simulink model "LaengsDynamicModell"  (R2018b)
settings: Solver=VariableStepAuto  StartTime=0.0  StopTime=10.0  RelTol=1e-3
model workspace (MAT data in the model file):
  g = 9.81
  hs = 0.5
  l = 2.8
  lv = 1.344
  rBreakPoints = [0 0.25 1]
  rBreakpoints = [0 0.25 1]
  rTableData = [0 1 1]
  v0 = 19.4444444444
  zBreakpoints = [0 1.5 1.95 2.15 10]
  zTableData = [0 0 0.1 1 1]
  zh_z = 1
  zv_z = 1
libraries: simulink x3
settings Model: Creator=User  LastModifiedBy=gregoryseibert

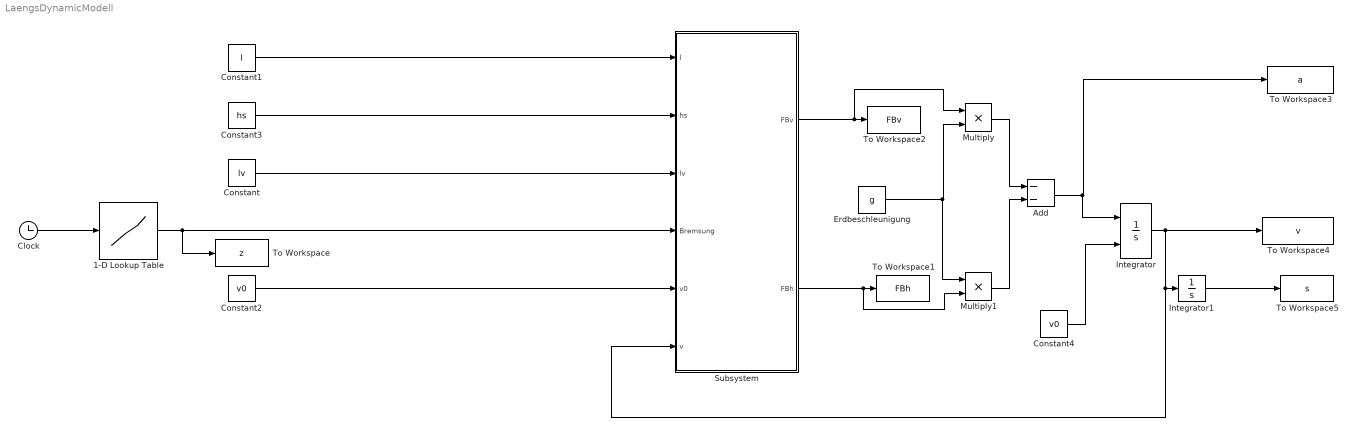
== system LaengsDynamicModell ==
  1-D Lookup Table : Lookup_n-D  NumberOfTableDimensions=1  BreakpointsForDimension1=zBreakpoints  Table=zTableData  InternalRulePriority=Speed  RndMeth=Simplest  InputSameDT=on
  Add : Sum  Inputs=--
  Clock : Clock
  Constant : Constant  Value=lv
  Constant1 : Constant  Value=l
  Constant2 : Constant  Value=v0
  Constant3 : Constant  Value=hs
  Constant4 : Constant  Value=v0
  "Erdbeschleunigung " : Constant  Value=g
  Integrator : Integrator  InitialConditionSource=external  LimitOutput=on  LowerSaturationLimit=0
  Integrator1 : Integrator
  Multiply : Product
  Multiply1 : Product
  Subsystem : Subsystem
  To Workspace : ToWorkspace  VariableName=z  SaveFormat=Timeseries  SampleTime=-1
  To Workspace1 : ToWorkspace  VariableName=FBh  SaveFormat=Timeseries  SampleTime=-1
  To Workspace2 : ToWorkspace  VariableName=FBv  SaveFormat=Timeseries  SampleTime=-1
  To Workspace3 : ToWorkspace  VariableName=a  SaveFormat=Timeseries  SampleTime=-1
  To Workspace4 : ToWorkspace  VariableName=v  SaveFormat=Timeseries  SampleTime=-1
  To Workspace5 : ToWorkspace  VariableName=s  SaveFormat=Timeseries  SampleTime=-1
  wires:
  Clock/1 -> 1-D Lookup Table/1
  1-D Lookup Table/1 -> Subsystem/4("Bremsung "), To Workspace/1
  Constant1/1 -> Subsystem/1("l ")
  Constant3/1 -> Subsystem/2(hs)
  Constant/1 -> Subsystem/3(lv)
  Constant2/1 -> Subsystem/5("v0 ")
  Subsystem/1(FBv) -> Multiply/1, To Workspace2/1
  Subsystem/2(FBh) -> Multiply1/2, To Workspace1/1
  "Erdbeschleunigung "/1 -> Multiply1/1, Multiply/2
  Multiply/1 -> Add/1
  Multiply1/1 -> Add/2
  Add/1 -> Integrator/1, To Workspace3/1
  Constant4/1 -> Integrator/2
  Integrator/1 -> Subsystem/6("v "), Integrator1/1, To Workspace4/1
  Integrator1/1 -> To Workspace5/1

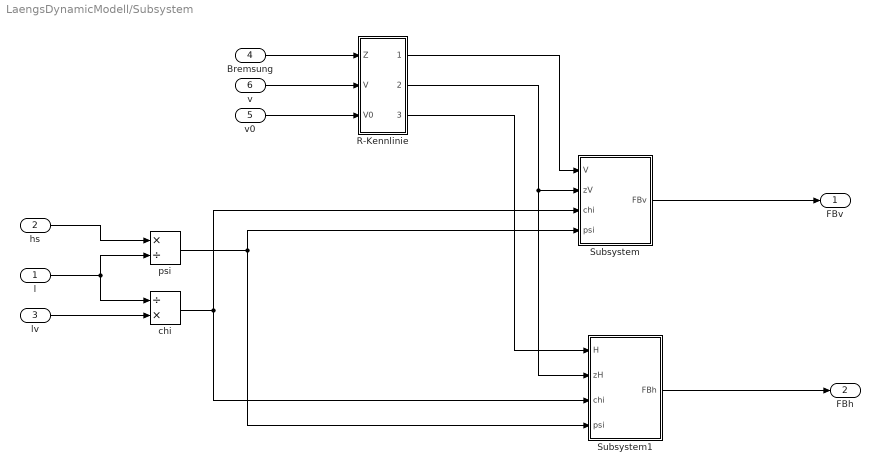
== system LaengsDynamicModell/Subsystem ==
  "l " : Inport
  hs : Inport  Port=2
  lv : Inport  Port=3
  "Bremsung " : Inport  Port=4
  "v0 " : Inport  Port=5
  "v " : Inport  Port=6
  R-Kennlinie : Subsystem
  Subsystem : Subsystem
  Subsystem1 : Subsystem
  chi : Product  Inputs=/*
  psi : Product  Inputs=*/
  FBv : Outport
  FBh : Outport  Port=2
  wires:
  "l "/1 -> chi/1, psi/2
  hs/1 -> psi/1
  lv/1 -> chi/2
  "Bremsung "/1 -> R-Kennlinie/1(Z)
  "v "/1 -> R-Kennlinie/2(V)
  "v0 "/1 -> R-Kennlinie/3("V0 ")
  psi/1 -> Subsystem/4(psi), Subsystem1/4(psi)
  chi/1 -> Subsystem/3(chi), Subsystem1/3(chi)
  R-Kennlinie/2("zOut ") -> Subsystem1/2(zH), Subsystem/2(zV)
  R-Kennlinie/3(hOut) -> Subsystem1/1(H)
  R-Kennlinie/1(vOut) -> Subsystem/1(V)
  Subsystem/1(FBv) -> FBv/1
  Subsystem1/1(FBh) -> FBh/1

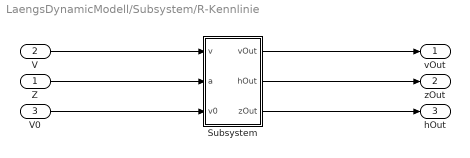
== system LaengsDynamicModell/Subsystem/R-Kennlinie ==
  Z : Inport
  V : Inport  Port=2
  "V0 " : Inport  Port=3
  Subsystem : Subsystem
  vOut : Outport
  "zOut " : Outport  Port=2
  hOut : Outport  Port=3
  wires:
  Z/1 -> Subsystem/2("a ")
  V/1 -> Subsystem/1(v)
  "V0 "/1 -> Subsystem/3(v0)
  Subsystem/3(zOut) -> hOut/1
  Subsystem/2(hOut) -> "zOut "/1
  Subsystem/1(vOut) -> vOut/1

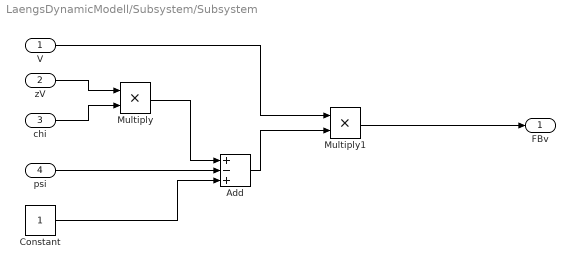
== system LaengsDynamicModell/Subsystem/Subsystem ==
  V : Inport
  zV : Inport  Port=2
  chi : Inport  Port=3
  psi : Inport  Port=4
  Add : Sum  Inputs=+-+
  Constant : Constant
  Multiply : Product
  Multiply1 : Product
  FBv : Outport
  wires:
  zV/1 -> Multiply/1
  chi/1 -> Multiply/2
  Multiply/1 -> Add/1
  psi/1 -> Add/2
  Constant/1 -> Add/3
  V/1 -> Multiply1/1
  Add/1 -> Multiply1/2
  Multiply1/1 -> FBv/1

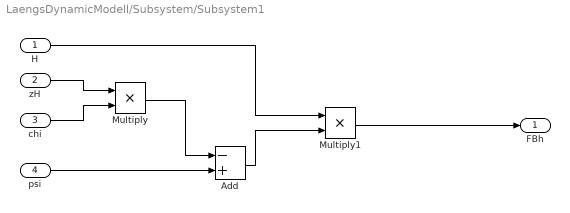
== system LaengsDynamicModell/Subsystem/Subsystem1 ==
  H : Inport
  zH : Inport  Port=2
  chi : Inport  Port=3
  psi : Inport  Port=4
  Add : Sum  Inputs=-+
  Multiply : Product
  Multiply1 : Product
  FBh : Outport
  wires:
  zH/1 -> Multiply/1
  chi/1 -> Multiply/2
  Multiply/1 -> Add/1
  psi/1 -> Add/2
  H/1 -> Multiply1/1
  Add/1 -> Multiply1/2
  Multiply1/1 -> FBh/1

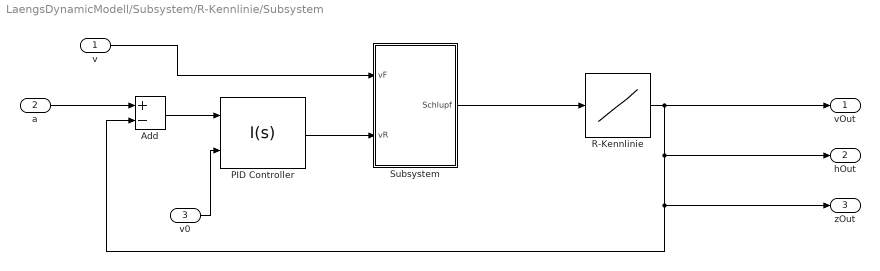
== system LaengsDynamicModell/Subsystem/R-Kennlinie/Subsystem ==
  v : Inport
  "a " : Inport  Port=2
  v0 : Inport  Port=3
  Add : Sum  Inputs=+-
  PID Controller : simulink/Continuous/PID Controller  Controller=I  Form=Parallel  TimeDomain=Continuous-time  SampleTime=-1  IntegratorMethod=Forward Euler  FilterMethod=Forward Euler  ControllerParametersSource=internal  P=1  I=-700  D=0  UseFilter=on  N=100  TunerSelectOption=Transfer Function Based (PID Tuner App)  InitialConditionSource=external  InitialConditionForIntegrator=0  InitialConditionForFilter=0  DifferentiatorICPrevScaledInput=0  ExternalReset=none  TrackingMode=off  Kt=1  LimitOutput=off  UpperSaturationLimit=inf  LowerSaturationLimit=-inf  LinearizeAsGain=on  AntiWindupMode=none  Kb=1  POutMin=[]  POutMax=[]  IOutMin=[]  IOutMax=[]  DOutMin=[]  DOutMax=[]  NOutMin=[]  NOutMax=[]  SumOutMin=[]  SumOutMax=[]  SaturationOutMin=[]  SaturationOutMax=[]  PParamMin=[]  PParamMax=[]  IParamMin=[]  IParamMax=[]  DParamMin=[]  DParamMax=[]  NParamMin=[]  NParamMax=[]  KbParamMin=[]  KbParamMax=[]  KtParamMin=[]  KtParamMax=[]  KbOutMin=[]  KbOutMax=[]  KtOutMin=[]  KtOutMax=[]  IntegratorOutMin=[]  IntegratorOutMax=[]  FilterOutMin=[]  FilterOutMax=[]  SumI1OutMin=[]  SumI1OutMax=[]  SumI2OutMin=[]  SumI2OutMax=[]  SumI3OutMin=[]  SumI3OutMax=[]  SumI4OutMin=[]  SumI4OutMax=[]  SumDOutMin=[]  SumDOutMax=[]  DifferentiatorOutMin=[]  DifferentiatorOutMax=[]  FilterDiffOutCoefMin=[]  FilterDiffOutCoefMax=[]  ReciprocalOutMin=[]  ReciprocalOutMax=[]  SumDenOutMin=[]  SumDenOutMax=[]  SumNumOutMin=[]  SumNumOutMax=[]  DivideOutMin=[]  DivideOutMax=[]  IntegratorContinuousStateAttributes=''  IntegratorStateMustResolveToSignalObject=off  IntegratorRTWStateStorageClass=Auto  FilterContinuousStateAttributes=''  FilterStateMustResolveToSignalObject=off  FilterRTWStateStorageClass=Auto  ParallelPVariant=Disabled  IdealPVariant=Disabled  IVariant=InternalParameters  DVariant=Disabled  IntegratorVariant=Continuous  SatVariant=Disabled  AWVariant=Passthrough  PCopyVariant=Disabled  TRVariant=Disabled  FdbkBlocksVariant=Forward  IdealPFdbkVariant=Disabled  SatFdbkVariant=Disabled  DerivativeFilterVariant=Disabled  NVariant=Disabled  NCopyVariant=Disabled_SignalSpec  FilterICVariant=Disabled  IntegratorICVariant=ExternalICs  ExternalResetVariant=Disabled  TRSumVariant=Passthrough  SumFdbkVariant=Disabled  SumVariant=Passthrough_I
  R-Kennlinie : Lookup_n-D  NumberOfTableDimensions=1  BreakpointsForDimension1=rBreakpoints  Table=rTableData  InternalRulePriority=Speed  RndMeth=Simplest  InputSameDT=on
  Subsystem : Subsystem
  vOut : Outport
  hOut : Outport  Port=2
  zOut : Outport  Port=3
  wires:
  v/1 -> Subsystem/1(vF)
  "a "/1 -> Add/1
  Add/1 -> PID Controller/1
  v0/1 -> PID Controller/2
  PID Controller/1 -> Subsystem/2("vR ")
  Subsystem/1("Schlupf ") -> R-Kennlinie/1
  R-Kennlinie/1 -> zOut/1, Add/2, hOut/1, vOut/1

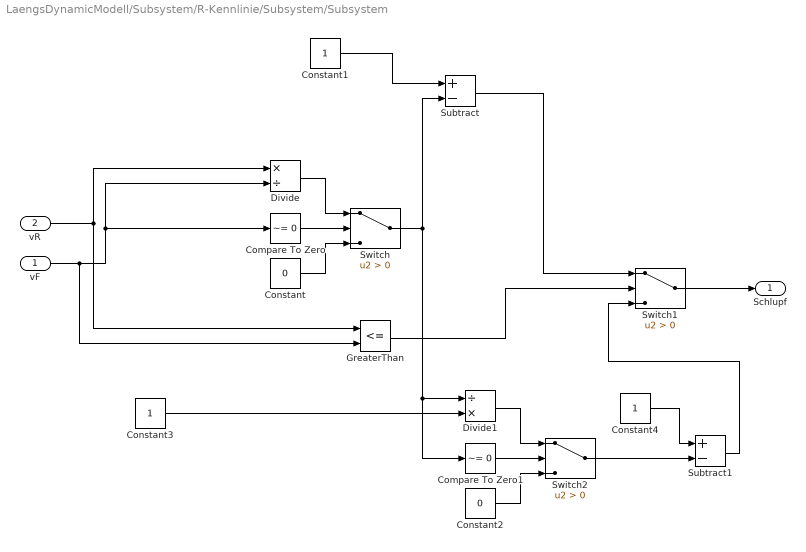
== system LaengsDynamicModell/Subsystem/R-Kennlinie/Subsystem/Subsystem ==
  vF : Inport
  "vR " : Inport  Port=2
  Compare To Zero : simulink/Logic and Bit Operations/Compare To Zero  relop=~=  OutDataTypeStr=boolean
  Compare To Zero1 : simulink/Logic and Bit Operations/Compare To Zero  relop=~=  OutDataTypeStr=boolean
  Constant : Constant  Value=0
  Constant1 : Constant
  Constant2 : Constant  Value=0
  Constant3 : Constant
  Constant4 : Constant
  Divide : Product  Inputs=*/
  Divide1 : Product  Inputs=/*
  GreaterThan : RelationalOperator  Operator=<=  OutDataTypeStr=boolean  RndMeth=Simplest
  Subtract : Sum  Inputs=+-
  Subtract1 : Sum  Inputs=+-
  Switch : Switch  Criteria=u2 > Threshold
  Switch1 : Switch  Criteria=u2 > Threshold
  Switch2 : Switch  Criteria=u2 > Threshold
  "Schlupf " : Outport
  wires:
  Compare To Zero/1 -> Switch/2
  Divide/1 -> Switch/1
  Constant/1 -> Switch/3
  "vR "/1 -> GreaterThan/1, Divide/1
  vF/1 -> GreaterThan/2, Divide/2, Compare To Zero/1
  Constant1/1 -> Subtract/1
  Switch/1 -> Divide1/1, Compare To Zero1/1, Subtract/2
  Subtract/1 -> Switch1/1
  GreaterThan/1 -> Switch1/2
  Switch1/1 -> "Schlupf "/1
  Divide1/1 -> Switch2/1
  Constant2/1 -> Switch2/3
  Compare To Zero1/1 -> Switch2/2
  Constant3/1 -> Divide1/2
  Switch2/1 -> Subtract1/2
  Constant4/1 -> Subtract1/1
  Subtract1/1 -> Switch1/3
